simulink library "vmc"  (R2021b)
settings: Solver=VariableStepAuto  StartTime=0.0  StopTime=10.0  RelTol=1e-3
undefined symbols (not defined in the file): AVMC_ACCDeltaTqGradeGn_X_deg, AVMC_ACCDeltaTqIGain4OVRD_X_kph, AVMC_ACCDeltaTqIGain4OVRD_Y_mps2, AVMC_ACCDeltaTqIGain_X_kph, AVMC_ACCDeltaTqIGain_Y_mps2, AVMC_ACCDeltaTqPGain_X_kph, AVMC_ACCDeltaTqPGain_Y_kph, AVMC_ACCGradeofst_X_G, AVMC_ACCGradeofst_Y_pct, AVMC_ACCLoSpdTqLoLim4JP_X_kph, AVMC_ACCLoSpdTqLoLim4JP_Y_deg, AVMC_ACCLoSpdTqLowerLim_X_kph, AVMC_ACCLoSpdTqLowerLim_Y_deg, AVMC_ACCReqAccelGain_X_mps2, AVMC_ACCReqAccelGain_Y_enum, AVMC_ADSPosGFBDeltaTq_X_kph, AVMC_ADSPosGFBDeltaTq_Y_mps2, AVMC_AggressJerkPCT4AT_X_kph, AVMC_AggressJerkPCT_X_kph, AVMC_AggressLimitPCT4AT_X_kph, AVMC_AggressLimitPCT_X_kph, AVMC_DECGradeofst_X_G, AVMC_DECGradeofst_Y_pct, AVMC_DISCDeltaTqIGain_X_kph, AVMC_DISCDeltaTqIGain_Y_mps2, AVMC_DISCDeltaTqPGain_X_kph, AVMC_DISCDeltaTqPGain_Y_kph, AVMC_EPSForceSelect_X_enum, AVMC_EPSForceSelect_Y_enum, AVMC_EPSForceSelectD21_X_enum, AVMC_EPSForceSelectD21_Y_enum, AVMC_ESCRegenOut_X_kph, AVMC_ESCRegenOut_Y_Deg, AVMC_ESCRegenOutEnSpd_X_Deg, AVMC_EstPitchSlopeTs_X_kph, AVMC_GradeCompFlt_X_kph, AVMC_GyroYBandLo_X_Gps, AVMC_HoldResTq_X_kph, AVMC_ISOAccLimit_X_mps, AVMC_ISODecLimit_X_mps, AVMC_ISOJerk_X_mps, AVMC_LatESCRegenOut_X_kph, AVMC_LatESCRegenOut_Y_Deg, AVMC_LongAccDeadZone_X_kph, AVMC_LongAccFiltTsforP2_X_Gps, AVMC_MCPresBaseTq_X_bar, AVMC_MSAPedalOvrd_X_kph, AVMC_MSASpdBand_X_kph, AVMC_MSATqDownEndTq_X_kph, AVMC_MSATqDownTime_X_kph, AVMC_NegZCHoldTq_X_kph, AVMC_OPDDisSlideRate_X_Deg, AVMC_OVRD2ActSR2FCMCMD_X_mps2, AVMC_PedalTqRWhlRatio_X_Nm, AVMC_PedalTqRWhlRatio_Y_gps, AVMC_PedalTqRWhlSlipGain_X_rat, AVMC_PedalTqRWhlSlipGain_Y_kph, AVMC_PedalTqRWhSTRGGain_X_deg, AVMC_PedalTqRWhSTRGGain_Y_kph, AVMC_PosZCHoldTq_X_kph ... (+593)
libraries: hcu_lib x143, simulink x96, tqr x4, $bdroot x1, simulink_extras x1
(part 17 of 17)

== stateflow chart vmc/VMC/VMC/SafetyControl/WheelSpeedRollingAverage/RollingAverage1 ==
  state LatAccelRollingAverage
    (default) -> (junction 2) : {VVMC_RollAveCount_enum = ONE_INT}
    LatAccelRollingAverage -> (junction 2)
    (junction 2) -> (junction 3) : {VVMC_RFWhlSpeedRollAveRaw_kph = ZERO_FLOAT}
    (junction 3) -> (junction 100) [order 1] : [VVMC_RollAveCount_enum < KVMC_WhlSpdRollAveLevel_enum]
    (junction 3) -> (junction 37) [order 2]
    (junction 100) -> (junction 5) : {% Memory
        |  VVMC_Memory_raw32[VVMC_RollAveCount_enum] = VINP_RFRawWhlSpeed_kph;
        |
        |  % Memory Shift Counter
        |  VVMC_ShiftCount_enum = ONE_INT}
    (junction 5) -> (junction 7) [order 2]
    (junction 5) -> (junction 6) [order 1] : [VVMC_ShiftCount_enum <= VVMC_RollAveCount_enum]
    (junction 7) -> (junction 8) : {% Rolling Average
        |  VVMC_RFWhlSpeedRollAveRaw_kph = VVMC_RFWhlSpeedRollAveRaw_kph / VVMC_RollAveCount_enum;
        |
        |  % Rolling Average Counter
        |  VVMC_RollAveCount_enum++}
    (junction 35) -> (junction 5) : {VVMC_ShiftCount_enum++}
    (junction 6) -> (junction 36) : {% Rolling Average Sum
        |  VVMC_RFWhlSpeedRollAveRaw_kph = VVMC_RFWhlSpeedRollAveRaw_kph + VVMC_Memory_raw32[VVMC_ShiftCount_enum];
        |  }
    (junction 36) -> (junction 35)
    (junction 37) -> (junction 76) [order 1] : [VVMC_RollAveCount_enum == KVMC_WhlSpdRollAveLevel_enum]
    (junction 76) -> (junction 47)
    (junction 37) -> (junction 60) [order 2]
    (junction 78) -> (junction 76)
    (junction 47) -> (junction 30) : {% Memory
        |  VVMC_Memory_raw32[VVMC_RollAveCount_enum] = VINP_RFRawWhlSpeed_kph;
        |
        |  % Memory Shift Counter
        |  VVMC_ShiftCount_enum = ONE_INT;
        | }
    (junction 60) -> (junction 62) [order 1] : [VVMC_RollAveCount_enum > KVMC_WhlSpdRollAveLevel_enum]
    (junction 60) -> (junction 39) [order 2]
    (junction 62) -> (junction 66) : {VVMC_MemoryShiftCount_enum = ONE_INT}
    (junction 30) -> (junction 48) [order 2]
    (junction 30) -> (junction 22) [order 1] : [VVMC_ShiftCount_enum <= VVMC_RollAveCount_enum]
    (junction 48) -> (junction 45) : {% Rolling Average
        |  VVMC_RFWhlSpeedRollAveRaw_kph = VVMC_RFWhlSpeedRollAveRaw_kph / VVMC_RollAveCount_enum;
        |
        |  % Memory Shift Counter
        |  VVMC_ShiftCount_enum = ONE_INT}
    (junction 14) -> (junction 30) : {VVMC_ShiftCount_enum++}
    (junction 22) -> (junction 25) : {% Rolling Average Sum
        |  VVMC_RFWhlSpeedRollAveRaw_kph = VVMC_RFWhlSpeedRollAveRaw_kph + VVMC_Memory_raw32[VVMC_ShiftCount_enum]}
    (junction 66) -> (junction 82) [order 2]
    (junction 66) -> (junction 69) [order 1] : [VVMC_MemoryShiftCount_enum < VVMC_RollAveCount_enum]
    (junction 82) -> (junction 80) : {VVMC_RollAveCount_enum = KVMC_WhlSpdRollAveLevel_enum}
    (junction 73) -> (junction 66) : {VVMC_MemoryShiftCount_enum++}
    (junction 69) -> (junction 71) : {VVMC_Memory_raw32[VVMC_MemoryShiftCount_enum] =...
        |  VVMC_Memory_raw32[VVMC_RollAveCount_enum - KVMC_WhlSpdRollAveLevel_enum + VVMC_MemoryShiftCount_enum]}
    (junction 25) -> (junction 14)
    (junction 71) -> (junction 73)
    (junction 80) -> (junction 78)
    (junction 45) -> (junction 39) [order 2]
    (junction 45) -> (junction 15) [order 1] : [VVMC_ShiftCount_enum < VVMC_RollAveCount_enum]
    (junction 41) -> (junction 45) : { VVMC_ShiftCount_enum++}
    (junction 15) -> (junction 38) : {% Gy Memory Shift
        |  VVMC_Memory_raw32[VVMC_ShiftCount_enum] = VVMC_Memory_raw32[VVMC_ShiftCount_enum + ONE_INT]}
    (junction 38) -> (junction 41)
  data: KVMC_WhlSpdRollAveLevel_enum input uint8; VVMC_ShiftCount_enum local uint8; VVMC_RollAveCount_enum local uint8; VVMC_Memory_raw32 local single size=256; ZERO_FLOAT input single; ONE_INT input uint8; VINP_RFRawWhlSpeed_kph input single; VVMC_MemoryShiftCount_enum local uint8; VVMC_RFWhlSpeedRollAveRaw_kph output single

== stateflow chart vmc/VMC/VMC/SafetyControl/WheelSpeedRollingAverage/RollingAverage2 ==
  state LatAccelRollingAverage
    (default) -> (junction 2) : {VVMC_RollAveCount_enum = ONE_INT}
    LatAccelRollingAverage -> (junction 2)
    (junction 2) -> (junction 3) : {VVMC_LRWhlSpeedRollAveRaw_kph = ZERO_FLOAT}
    (junction 3) -> (junction 100) [order 1] : [VVMC_RollAveCount_enum < KVMC_WhlSpdRollAveLevel_enum]
    (junction 3) -> (junction 37) [order 2]
    (junction 100) -> (junction 5) : {% Memory
        |  VVMC_Memory_raw32[VVMC_RollAveCount_enum] = VINP_LRRawWhlSpeed_kph;
        |
        |  % Memory Shift Counter
        |  VVMC_ShiftCount_enum = ONE_INT}
    (junction 5) -> (junction 7) [order 2]
    (junction 5) -> (junction 6) [order 1] : [VVMC_ShiftCount_enum <= VVMC_RollAveCount_enum]
    (junction 7) -> (junction 8) : {% Rolling Average
        |  VVMC_LRWhlSpeedRollAveRaw_kph = VVMC_LRWhlSpeedRollAveRaw_kph / VVMC_RollAveCount_enum;
        |
        |  % Rolling Average Counter
        |  VVMC_RollAveCount_enum++}
    (junction 35) -> (junction 5) : {VVMC_ShiftCount_enum++}
    (junction 6) -> (junction 36) : {% Rolling Average Sum
        |  VVMC_LRWhlSpeedRollAveRaw_kph = VVMC_LRWhlSpeedRollAveRaw_kph + VVMC_Memory_raw32[VVMC_ShiftCount_enum];
        |  }
    (junction 36) -> (junction 35)
    (junction 37) -> (junction 76) [order 1] : [VVMC_RollAveCount_enum == KVMC_WhlSpdRollAveLevel_enum]
    (junction 76) -> (junction 47)
    (junction 37) -> (junction 60) [order 2]
    (junction 78) -> (junction 76)
    (junction 47) -> (junction 30) : {% Memory
        |  VVMC_Memory_raw32[VVMC_RollAveCount_enum] = VINP_LRRawWhlSpeed_kph;
        |
        |  % Memory Shift Counter
        |  VVMC_ShiftCount_enum = ONE_INT;
        | }
    (junction 60) -> (junction 62) [order 1] : [VVMC_RollAveCount_enum > KVMC_WhlSpdRollAveLevel_enum]
    (junction 60) -> (junction 39) [order 2]
    (junction 62) -> (junction 66) : {VVMC_MemoryShiftCount_enum = ONE_INT}
    (junction 30) -> (junction 48) [order 2]
    (junction 30) -> (junction 22) [order 1] : [VVMC_ShiftCount_enum <= VVMC_RollAveCount_enum]
    (junction 48) -> (junction 45) : {% Rolling Average
        |  VVMC_LRWhlSpeedRollAveRaw_kph = VVMC_LRWhlSpeedRollAveRaw_kph / VVMC_RollAveCount_enum;
        |
        |  % Memory Shift Counter
        |  VVMC_ShiftCount_enum = ONE_INT}
    (junction 14) -> (junction 30) : {VVMC_ShiftCount_enum++}
    (junction 22) -> (junction 25) : {% Rolling Average Sum
        |  VVMC_LRWhlSpeedRollAveRaw_kph = VVMC_LRWhlSpeedRollAveRaw_kph + VVMC_Memory_raw32[VVMC_ShiftCount_enum]}
    (junction 66) -> (junction 82) [order 2]
    (junction 66) -> (junction 69) [order 1] : [VVMC_MemoryShiftCount_enum < VVMC_RollAveCount_enum]
    (junction 82) -> (junction 80) : {VVMC_RollAveCount_enum = KVMC_WhlSpdRollAveLevel_enum}
    (junction 73) -> (junction 66) : {VVMC_MemoryShiftCount_enum++}
    (junction 69) -> (junction 71) : {VVMC_Memory_raw32[VVMC_MemoryShiftCount_enum] =...
        |  VVMC_Memory_raw32[VVMC_RollAveCount_enum - KVMC_WhlSpdRollAveLevel_enum + VVMC_MemoryShiftCount_enum]}
    (junction 25) -> (junction 14)
    (junction 71) -> (junction 73)
    (junction 80) -> (junction 78)
    (junction 45) -> (junction 39) [order 2]
    (junction 45) -> (junction 15) [order 1] : [VVMC_ShiftCount_enum < VVMC_RollAveCount_enum]
    (junction 41) -> (junction 45) : { VVMC_ShiftCount_enum++}
    (junction 15) -> (junction 38) : {% Gy Memory Shift
        |  VVMC_Memory_raw32[VVMC_ShiftCount_enum] = VVMC_Memory_raw32[VVMC_ShiftCount_enum + ONE_INT]}
    (junction 38) -> (junction 41)
  data: KVMC_WhlSpdRollAveLevel_enum input uint8; VVMC_ShiftCount_enum local uint8; VVMC_RollAveCount_enum local uint8; VVMC_Memory_raw32 local single size=256; ZERO_FLOAT input single; ONE_INT input uint8; VINP_LRRawWhlSpeed_kph input single; VVMC_MemoryShiftCount_enum local uint8; VVMC_LRWhlSpeedRollAveRaw_kph output single

== stateflow chart vmc/VMC/VMC/SafetyControl/WheelSpeedRollingAverage/RollingAverage3 ==
  state LatAccelRollingAverage
    (default) -> (junction 2) : {VVMC_RollAveCount_enum = ONE_INT}
    LatAccelRollingAverage -> (junction 2)
    (junction 2) -> (junction 3) : {VVMC_RRWhlSpeedRollAveRaw_kph = ZERO_FLOAT}
    (junction 3) -> (junction 100) [order 1] : [VVMC_RollAveCount_enum < KVMC_WhlSpdRollAveLevel_enum]
    (junction 3) -> (junction 37) [order 2]
    (junction 100) -> (junction 5) : {% Memory
        |  VVMC_Memory_raw32[VVMC_RollAveCount_enum] = VINP_RRRawWhlSpeed_kph;
        |
        |  % Memory Shift Counter
        |  VVMC_ShiftCount_enum = ONE_INT}
    (junction 5) -> (junction 7) [order 2]
    (junction 5) -> (junction 6) [order 1] : [VVMC_ShiftCount_enum <= VVMC_RollAveCount_enum]
    (junction 7) -> (junction 8) : {% Rolling Average
        |  VVMC_RRWhlSpeedRollAveRaw_kph = VVMC_RRWhlSpeedRollAveRaw_kph / VVMC_RollAveCount_enum;
        |
        |  % Rolling Average Counter
        |  VVMC_RollAveCount_enum++}
    (junction 35) -> (junction 5) : {VVMC_ShiftCount_enum++}
    (junction 6) -> (junction 36) : {% Rolling Average Sum
        |  VVMC_RRWhlSpeedRollAveRaw_kph = VVMC_RRWhlSpeedRollAveRaw_kph + VVMC_Memory_raw32[VVMC_ShiftCount_enum];
        |  }
    (junction 36) -> (junction 35)
    (junction 37) -> (junction 76) [order 1] : [VVMC_RollAveCount_enum == KVMC_WhlSpdRollAveLevel_enum]
    (junction 76) -> (junction 47)
    (junction 37) -> (junction 60) [order 2]
    (junction 78) -> (junction 76)
    (junction 47) -> (junction 30) : {% Memory
        |  VVMC_Memory_raw32[VVMC_RollAveCount_enum] = VINP_RRRawWhlSpeed_kph;
        |
        |  % Memory Shift Counter
        |  VVMC_ShiftCount_enum = ONE_INT;
        | }
    (junction 60) -> (junction 62) [order 1] : [VVMC_RollAveCount_enum > KVMC_WhlSpdRollAveLevel_enum]
    (junction 60) -> (junction 39) [order 2]
    (junction 62) -> (junction 66) : {VVMC_MemoryShiftCount_enum = ONE_INT}
    (junction 30) -> (junction 48) [order 2]
    (junction 30) -> (junction 22) [order 1] : [VVMC_ShiftCount_enum <= VVMC_RollAveCount_enum]
    (junction 48) -> (junction 45) : {% Rolling Average
        |  VVMC_RRWhlSpeedRollAveRaw_kph = VVMC_RRWhlSpeedRollAveRaw_kph / VVMC_RollAveCount_enum;
        |
        |  % Memory Shift Counter
        |  VVMC_ShiftCount_enum = ONE_INT}
    (junction 14) -> (junction 30) : {VVMC_ShiftCount_enum++}
    (junction 22) -> (junction 25) : {% Rolling Average Sum
        |  VVMC_RRWhlSpeedRollAveRaw_kph = VVMC_RRWhlSpeedRollAveRaw_kph + VVMC_Memory_raw32[VVMC_ShiftCount_enum]}
    (junction 66) -> (junction 82) [order 2]
    (junction 66) -> (junction 69) [order 1] : [VVMC_MemoryShiftCount_enum < VVMC_RollAveCount_enum]
    (junction 82) -> (junction 80) : {VVMC_RollAveCount_enum = KVMC_WhlSpdRollAveLevel_enum}
    (junction 73) -> (junction 66) : {VVMC_MemoryShiftCount_enum++}
    (junction 69) -> (junction 71) : {VVMC_Memory_raw32[VVMC_MemoryShiftCount_enum] =...
        |  VVMC_Memory_raw32[VVMC_RollAveCount_enum - KVMC_WhlSpdRollAveLevel_enum + VVMC_MemoryShiftCount_enum]}
    (junction 25) -> (junction 14)
    (junction 71) -> (junction 73)
    (junction 80) -> (junction 78)
    (junction 45) -> (junction 39) [order 2]
    (junction 45) -> (junction 15) [order 1] : [VVMC_ShiftCount_enum < VVMC_RollAveCount_enum]
    (junction 41) -> (junction 45) : { VVMC_ShiftCount_enum++}
    (junction 15) -> (junction 38) : {% Gy Memory Shift
        |  VVMC_Memory_raw32[VVMC_ShiftCount_enum] = VVMC_Memory_raw32[VVMC_ShiftCount_enum + ONE_INT]}
    (junction 38) -> (junction 41)
  data: KVMC_WhlSpdRollAveLevel_enum input uint8; VVMC_ShiftCount_enum local uint8; VVMC_RollAveCount_enum local uint8; VVMC_Memory_raw32 local single size=256; ZERO_FLOAT input single; ONE_INT input uint8; VINP_RRRawWhlSpeed_kph input single; VVMC_MemoryShiftCount_enum local uint8; VVMC_RRWhlSpeedRollAveRaw_kph output single

== stateflow chart vmc/VMC/VMC/Scheduler ==
  state Scheduler
    (default) -> (junction 3) : {counter = 0;}
    Scheduler -> (junction 3) : {counter++}
    (junction 3) -> (junction 5) [order 1] : [counter%%2 == 0]
    (junction 3) -> (junction 11) [order 2]
    (junction 5) -> (junction 7) : {Trigger_10ms_1;
        |  counter = 0;}
    (junction 7) -> (junction 11)
  data: counter local uint8
  events: Trigger_10ms_1 output FUNCTION_CALL_EVENT

== stateflow chart vmc/VMC/VMC/SpeedArbitration/Feature Arbitration/Feature Arbitration ==
  state FeatureArbitration
    (default) -> (junction 406) : {VVMC_FeatArbitrSta_enum = ENUM_FEATARBITRSTA_INACTIVE;
        |  VVMC_FeatReqSpd_kph = ZERO_FLOAT;}
    FeatureArbitration -> (junction 406)
    (junction 406) -> (junction 409) [order 1] : [VVMC_FeatStaConfirm_enum == ENUM_FEATSTACFM_AEB]
    (junction 406) -> (junction 413) [order 2]
    (junction 409) -> (junction 411) : {VVMC_FeatArbitrSta_enum = ENUM_FEATARBITRSTA_AEB;
        |  VVMC_FeatReqSpd_kph = ZERO_FLOAT}
    (junction 413) -> (junction 415) [order 1] : [VVMC_FeatStaConfirm_enum == ENUM_FEATSTACFM_ACC]
    (junction 413) -> (junction 430) [order 2]
    (junction 415) -> (junction 417) : {VVMC_FeatArbitrSta_enum = ENUM_FEATARBITRSTA_ACC;
        |  VVMC_FeatReqSpd_kph = ZERO_FLOAT}
    (junction 430) -> (junction 431) [order 1] : [VVMC_FeatStaConfirm_enum == ENUM_FEATSTACFM_CC]
    (junction 430) -> (junction 440) [order 2]
    (junction 431) -> (junction 433) : {VVMC_FeatArbitrSta_enum = ENUM_FEATARBITRSTA_CC;
        |  VVMC_FeatReqSpd_kph = VVMC_FeatSetSpdForCalcu_kph}
    (junction 440) -> (junction 441) [order 1] : [VVMC_FeatStaConfirm_enum == ENUM_FEATSTACFM_DISC]
    (junction 440) -> (junction 445) [order 2]
    (junction 441) -> (junction 438) : {VVMC_FeatArbitrSta_enum = ENUM_FEATARBITRSTA_DISC;
        |  VVMC_FeatReqSpd_kph = VDSC_DISCTargetSpd_kph}
    (junction 445) -> (junction 443) [order 1] : [VVMC_FeatStaConfirm_enum == ENUM_FEATSTACFM_MSA]
    (junction 445) -> (junction 449) [order 2]
    (junction 443) -> (junction 444) : {VVMC_FeatArbitrSta_enum = ENUM_FEATARBITRSTA_MSA;
        |  VVMC_FeatReqSpd_kph = VVMC_FeatSetSpdForCalcu_kph}
    (junction 449) -> (junction 450) [order 1] : [VVMC_FeatStaConfirm_enum == ENUM_FEATSTACFM_ACCDISC]
    (junction 450) -> (junction 557) [order 1] : [VVMC_FeatSetSpdForCalcu_kph < VDSC_DISCTargetSpd_kph &&...
        |  !VDSC_PreACC_flg]
    (junction 449) -> (junction 512) [order 2]
    (junction 450) -> (junction 467) [order 2] : {VVMC_FeatArbitrSta_enum = ENUM_FEATARBITRSTA_ACCDISC;
        |  VVMC_FeatReqSpd_kph = VDSC_DISCTargetSpd_kph}
    (junction 557) -> (junction 553) : {VVMC_FeatArbitrSta_enum = ENUM_FEATARBITRSTA_ACC;
        |  VVMC_FeatReqSpd_kph = ZERO_FLOAT}
    (junction 512) -> (junction 514) [order 1] : [VVMC_FeatStaConfirm_enum == ENUM_FEATSTACFM_CCDISC ||...
        |  VVMC_FeatStaConfirm_enum == ENUM_FEATSTACFM_DISCMSA]
    (junction 514) -> (junction 516) [order 1] : [VVMC_FeatSetSpdForCalcu_kph < VDSC_DISCTargetSpd_kph]
    (junction 516) -> (junction 518) [order 1] : [VVMC_FeatStaConfirm_enum == ENUM_FEATSTACFM_CCDISC]
    (junction 512) -> (junction 527) [order 2] : {VVMC_FeatArbitrSta_enum = ENUM_FEATARBITRSTA_INACTIVE;
        |  VVMC_FeatReqSpd_kph = ZERO_FLOAT}
    (junction 514) -> (junction 525) [order 2] : {VVMC_FeatArbitrSta_enum = ENUM_FEATARBITRSTA_DISC;
        |  VVMC_FeatReqSpd_kph = VDSC_DISCTargetSpd_kph}
    (junction 516) -> (junction 522) [order 2] : {VVMC_FeatArbitrSta_enum = ENUM_FEATARBITRSTA_MSA;
        |  VVMC_FeatReqSpd_kph = VVMC_FeatSetSpdForCalcu_kph}
    (junction 518) -> (junction 520) : {VVMC_FeatArbitrSta_enum = ENUM_FEATARBITRSTA_CC;
        |  VVMC_FeatReqSpd_kph = VVMC_FeatSetSpdForCalcu_kph}
  data: VVMC_FeatStaConfirm_enum input uint8; VDSC_DISCTargetSpd_kph input single; VVMC_FeatSetSpdForCalcu_kph input single; VVMC_FeatArbitrSta_enum output uint8; VVMC_FeatReqSpd_kph output single; ENUM_FEATSTACFM_AEB input uint8; ENUM_FEATSTACFM_ACC input uint8; ENUM_FEATSTACFM_CC input uint8; ENUM_FEATSTACFM_DISC input uint8; ENUM_FEATSTACFM_MSA input uint8; ENUM_FEATSTACFM_ACCDISC input uint8; ENUM_FEATSTACFM_CCDISC input uint8; ENUM_FEATSTACFM_DISCMSA input uint8; ENUM_FEATARBITRSTA_INACTIVE input uint8; ENUM_FEATARBITRSTA_AEB input uint8; ENUM_FEATARBITRSTA_ACC input uint8; ENUM_FEATARBITRSTA_CC input uint8; ENUM_FEATARBITRSTA_DISC input uint8; ENUM_FEATARBITRSTA_ACCDISC input uint8; ENUM_FEATARBITRSTA_MSA input uint8; ZERO_FLOAT input single; VDSC_PreACC_flg input

== stateflow chart vmc/VMC/VMC/SpeedArbitration/Feature Status Confirm/Feature Status Confirm ==
  state FeatStaConfrim
    (default) -> (junction 197) : {VVMC_FeatStaConfirm_enum = ENUM_FEATSTACFM_INACTIVE}
    FeatStaConfrim -> (junction 197)
    (junction 197) -> (junction 203) [order 1] : [VVMC_VMCAEBCtrlAvail_flg == ENUM_VMCAEBCTRLAVAIL_AVAILABLE &&...
        | (VINP_ADASAEBSta_enum == ENUM_ADASAEBSTA_ACTIVE ||...
        |  VINP_ADASAEBReq_enum ~= ENUM_ADASAEBREQ_NOREQUEST)]
    (junction 197) -> (junction 200) [order 2]
    (junction 203) -> (junction 202) : {VVMC_FeatStaConfirm_enum = ENUM_FEATSTACFM_AEB}
    (junction 200) -> (junction 208) [order 1] : [VVMC_VMCACCCtrlAvail_flg == ENUM_VMCACCCTRLAVAIL_AVAILABLE &&...
        | (VDSC_DISCSta_enum == ENUM_DISCSTA_ACTIVE || VDSC_PreACC_flg)]
    (junction 208) -> (junction 210) [order 1] : [VINP_ADASACCSta_enum == ENUM_ADASACCSTA_ACTIVE ||...
        |  VINP_ADASACCSta_enum == ENUM_ADASACCSTA_SHUTOFF ||...
        |  VINP_ADASACCSta_enum == ENUM_ADASACCSTA_OVERRIDE]
    (junction 200) -> (junction 232) [order 2]
    (junction 208) -> (junction 214) [order 2]
    (junction 210) -> (junction 212) : {VVMC_FeatStaConfirm_enum = ENUM_FEATSTACFM_ACCDISC}
    (junction 214) -> (junction 216) [order 1] : [(VVMC_CCCtrlSta_enum == ENUM_CCCRLSTA_ACTIVE ||...
        |   VVMC_CCCtrlSta_enum == ENUM_CCCRLSTA_OVERRIDE) &&...
        |  VVMC_VMCCCCtrlAvail_flg == ENUM_VMCCCCTRLAVAIL_AVAILABLE]
    (junction 214) -> (junction 222) [order 2]
    (junction 216) -> (junction 218) : {VVMC_FeatStaConfirm_enum = ENUM_FEATSTACFM_CCDISC}
    (junction 222) -> (junction 224) [order 1] : [(VVMC_MSACtrlSta_enum == ENUM_MSACRLSTA_ACTIVE ||...
        |   VVMC_MSACtrlSta_enum == ENUM_MSACRLSTA_OVERRIDE) &&...
        |  VVMC_VMCMSACtrlAvail_flg == ENUM_VMCMSACTRLAVAIL_AVAILABLE]
    (junction 222) -> (junction 229) [order 2] : {VVMC_FeatStaConfirm_enum = ENUM_FEATSTACFM_DISC}
    (junction 224) -> (junction 221) : {VVMC_FeatStaConfirm_enum = ENUM_FEATSTACFM_DISCMSA}
    (junction 232) -> (junction 234) [order 1] : [VVMC_VMCACCCtrlAvail_flg == ENUM_VMCACCCTRLAVAIL_AVAILABLE &&...
        | (VINP_ADASACCSta_enum == ENUM_ADASACCSTA_ACTIVE ||...
        |  VINP_ADASACCSta_enum == ENUM_ADASACCSTA_OVERRIDE ||...
        |  VINP_ADASACCSta_enum == ENUM_ADASACCSTA_SHUTOFF)]
    (junction 232) -> (junction 238) [order 2]
    (junction 234) -> (junction 236) : {VVMC_FeatStaConfirm_enum = ENUM_FEATSTACFM_ACC}
    (junction 238) -> (junction 240) [order 1] : [(VVMC_CCCtrlSta_enum == ENUM_CCCRLSTA_ACTIVE ||...
        |   VVMC_CCCtrlSta_enum == ENUM_CCCRLSTA_OVERRIDE) &&...
        |  VVMC_VMCCCCtrlAvail_flg == ENUM_VMCCCCTRLAVAIL_AVAILABLE]
    (junction 238) -> (junction 250) [order 2]
    (junction 240) -> (junction 244) : {VVMC_FeatStaConfirm_enum = ENUM_FEATSTACFM_CC}
    (junction 250) -> (junction 249) [order 1] : [(VVMC_MSACtrlSta_enum == ENUM_MSACRLSTA_ACTIVE ||...
        |   VVMC_MSACtrlSta_enum == ENUM_MSACRLSTA_OVERRIDE) &&...
        |  VVMC_VMCMSACtrlAvail_flg == ENUM_VMCMSACTRLAVAIL_AVAILABLE]
    (junction 250) -> (junction 252) [order 2] : {VVMC_FeatStaConfirm_enum = ENUM_FEATSTACFM_INACTIVE}
    (junction 249) -> (junction 248) : {VVMC_FeatStaConfirm_enum = ENUM_FEATSTACFM_MSA}
  data: VVMC_VMCCCCtrlAvail_flg input boolean; ENUM_VMCCCCTRLAVAIL_AVAILABLE input uint8; VVMC_VMCMSACtrlAvail_flg input boolean; ENUM_VMCMSACTRLAVAIL_AVAILABLE input uint8; VVMC_VMCAEBCtrlAvail_flg input boolean; ENUM_VMCAEBCTRLAVAIL_AVAILABLE input uint8; VVMC_VMCACCCtrlAvail_flg input boolean; ENUM_VMCACCCTRLAVAIL_AVAILABLE input uint8; VINP_ADASAEBSta_enum input uint8; VDSC_DISCSta_enum input uint8; VINP_ADASACCSta_enum input uint8; VVMC_CCCtrlSta_enum input uint8; VVMC_FeatStaConfirm_enum output uint8; VVMC_MSACtrlSta_enum input uint8; ENUM_FEATSTACFM_INACTIVE input uint8; ENUM_FEATSTACFM_AEB input uint8; ENUM_FEATSTACFM_ACC input uint8; ENUM_FEATSTACFM_CC input uint8; ENUM_FEATSTACFM_DISC input uint8; ENUM_FEATSTACFM_MSA input uint8; ENUM_FEATSTACFM_ACCDISC input uint8; ENUM_FEATSTACFM_CCDISC input uint8; ENUM_FEATSTACFM_DISCMSA input uint8; ENUM_ADASAEBSTA_ACTIVE input uint8; ENUM_ADASACCSTA_ACTIVE input uint8; ENUM_ADASACCSTA_SHUTOFF input uint8; ENUM_CCCRLSTA_ACTIVE input uint8; ENUM_MSACRLSTA_ACTIVE input uint8; ENUM_DISCSTA_ACTIVE input uint8; ENUM_ADASACCSTA_OVERRIDE input uint8; VINP_ADASAEBReq_enum input uint8; ENUM_ADASAEBREQ_NOREQUEST input uint8; ENUM_CCCRLSTA_OVERRIDE input; ENUM_MSACRLSTA_OVERRIDE input; VDSC_PreACC_flg input

== stateflow chart vmc/VMC/VMC/SpeedArbitration/Response Gain/Response Gain ==
  state ResponseGain
    (default) -> (junction 81) : {VVMC_JerkPCT_pct = ZERO_FLOAT;
        |  VVMC_LimitPCT_pct = ZERO_FLOAT}
    ResponseGain -> (junction 81)
    (junction 81) -> (junction 73) [order 1] : [VVMC_FeatArbitrSta_enum == ENUM_FEATARBITRSTA_DISC ||...
        |  VVMC_FeatArbitrSta_enum == ENUM_FEATARBITRSTA_CC ||...
        |  VVMC_FeatArbitrSta_enum == ENUM_FEATARBITRSTA_MSA ||...
        |  VVMC_FeatArbitrSta_enum == ENUM_FEATARBITRSTA_ACCDISC]
    (junction 73) -> (junction 75) [order 1] : [VDSC_DISCTurn_flg == ENUM_DISCTURN_ACTIVE ||...
        | (VVMC_FeatArbitrSta_enum == ENUM_FEATARBITRSTA_MSA &&...
        |  KVMC_MSAResponseAGSV_flg == TRUE)]
    (junction 81) -> (junction 92) [order 2] : {VVMC_JerkPCT_pct = ZERO_FLOAT;
        |  VVMC_LimitPCT_pct = ZERO_FLOAT}
    (junction 73) -> (junction 77) [order 2] : {VVMC_JerkPCT_pct = VVMC_SoftJerkPCT_pct;
        |  VVMC_LimitPCT_pct = VVMC_SoftLimitPCT_pct}
    (junction 75) -> (junction 78) : {VVMC_JerkPCT_pct = VVMC_AggressJerkPCT_pct;
        |  VVMC_LimitPCT_pct = VVMC_AggressLimitPCT_pct}
  data: VDSC_DISCTurn_flg input uint8; VVMC_FeatArbitrSta_enum input uint8; VVMC_JerkPCT_pct output single; VVMC_LimitPCT_pct output single; VVMC_SoftJerkPCT_pct input single; VVMC_AggressJerkPCT_pct input single; VVMC_SoftLimitPCT_pct input single; VVMC_AggressLimitPCT_pct input single; ENUM_FEATARBITRSTA_DISC input uint8; ENUM_FEATARBITRSTA_CC input; ZERO_FLOAT input single; ENUM_DISCTURN_ACTIVE input uint8; ENUM_FEATARBITRSTA_ACCDISC input uint8; ENUM_FEATARBITRSTA_MSA input; TRUE input; KVMC_MSAResponseAGSV_flg input; ENUM_FEATARBITRSTA_ACC parameter

== stateflow chart vmc/VMC/VMC/SpeedCalculation/RollingAverage ==
  state LatAccelRollingAverage
    (default) -> (junction 2) : {VVMC_RollAveCount_enum = ONE_INT}
    LatAccelRollingAverage -> (junction 2)
    (junction 2) -> (junction 3) : {VVMC_RollAve_kph = ZERO_FLOAT}
    (junction 3) -> (junction 100) [order 1] : [VVMC_RollAveCount_enum < KVMC_RollAveLevel_enum]
    (junction 3) -> (junction 37) [order 2]
    (junction 100) -> (junction 5) : {% Memory
        |  VVMC_Memory_raw32[VVMC_RollAveCount_enum] = VINP_RawData_kph;
        |
        |  % Memory Shift Counter
        |  VVMC_ShiftCount_enum = ONE_INT}
    (junction 5) -> (junction 7) [order 2]
    (junction 5) -> (junction 6) [order 1] : [VVMC_ShiftCount_enum <= VVMC_RollAveCount_enum]
    (junction 7) -> (junction 8) : {% Rolling Average
        |  VVMC_RollAve_kph = VVMC_RollAve_kph / VVMC_RollAveCount_enum;
        |
        |  % Rolling Average Counter
        |  VVMC_RollAveCount_enum++}
    (junction 35) -> (junction 5) : {VVMC_ShiftCount_enum++}
    (junction 6) -> (junction 36) : {% Rolling Average Sum
        |  VVMC_RollAve_kph = VVMC_RollAve_kph + VVMC_Memory_raw32[VVMC_ShiftCount_enum];
        |  }
    (junction 36) -> (junction 35)
    (junction 37) -> (junction 76) [order 1] : [VVMC_RollAveCount_enum == KVMC_RollAveLevel_enum]
    (junction 76) -> (junction 47)
    (junction 37) -> (junction 60) [order 2]
    (junction 78) -> (junction 76)
    (junction 47) -> (junction 30) : {% Memory
        |  VVMC_Memory_raw32[VVMC_RollAveCount_enum] = VINP_RawData_kph;
        |
        |  % Memory Shift Counter
        |  VVMC_ShiftCount_enum = ONE_INT;
        | }
    (junction 60) -> (junction 62) [order 1] : [VVMC_RollAveCount_enum > KVMC_RollAveLevel_enum]
    (junction 60) -> (junction 39) [order 2]
    (junction 62) -> (junction 66) : {VVMC_MemoryShiftCount_enum = ONE_INT}
    (junction 30) -> (junction 48) [order 2]
    (junction 30) -> (junction 22) [order 1] : [VVMC_ShiftCount_enum <= VVMC_RollAveCount_enum]
    (junction 48) -> (junction 45) : {% Rolling Average
        |  VVMC_RollAve_kph = VVMC_RollAve_kph / VVMC_RollAveCount_enum;
        |
        |  % Memory Shift Counter
        |  VVMC_ShiftCount_enum = ONE_INT}
    (junction 14) -> (junction 30) : {VVMC_ShiftCount_enum++}
    (junction 22) -> (junction 25) : {% Rolling Average Sum
        |  VVMC_RollAve_kph = VVMC_RollAve_kph + VVMC_Memory_raw32[VVMC_ShiftCount_enum]}
    (junction 66) -> (junction 82) [order 2]
    (junction 66) -> (junction 69) [order 1] : [VVMC_MemoryShiftCount_enum < VVMC_RollAveCount_enum]
    (junction 82) -> (junction 80) : {VVMC_RollAveCount_enum = KVMC_RollAveLevel_enum}
    (junction 73) -> (junction 66) : {VVMC_MemoryShiftCount_enum++}
    (junction 69) -> (junction 71) : {VVMC_Memory_raw32[VVMC_MemoryShiftCount_enum] =...
        |  VVMC_Memory_raw32[VVMC_RollAveCount_enum - KVMC_RollAveLevel_enum + VVMC_MemoryShiftCount_enum]}
    (junction 25) -> (junction 14)
    (junction 71) -> (junction 73)
    (junction 80) -> (junction 78)
    (junction 45) -> (junction 39) [order 2]
    (junction 45) -> (junction 15) [order 1] : [VVMC_ShiftCount_enum < VVMC_RollAveCount_enum]
    (junction 41) -> (junction 45) : { VVMC_ShiftCount_enum++}
    (junction 15) -> (junction 38) : {% Gy Memory Shift
        |  VVMC_Memory_raw32[VVMC_ShiftCount_enum] = VVMC_Memory_raw32[VVMC_ShiftCount_enum + ONE_INT]}
    (junction 38) -> (junction 41)
  data: KVMC_RollAveLevel_enum input uint8; VVMC_ShiftCount_enum local uint8; VVMC_RollAveCount_enum local uint8; VVMC_Memory_raw32 local single size=256; ZERO_FLOAT input single; ONE_INT input uint8; VVMC_RollAve_kph output single; VINP_RawData_kph input single; VVMC_MemoryShiftCount_enum local uint8

== stateflow chart vmc/VMC/VMC/Scheduler1 ==
  state Scheduler
    (default) -> (junction 3) : {counter = 0;}
    Scheduler -> (junction 3) : {counter++}
    (junction 3) -> (junction 5) [order 1] : [counter%%2 == 0]
    (junction 3) -> (junction 11) [order 2]
    (junction 5) -> (junction 7) : {Trigger_LongAccel;
        |  counter = 0;}
    (junction 7) -> (junction 11)
  data: counter local uint8
  events: Trigger_LongAccel output FUNCTION_CALL_EVENT

== stateflow chart vmc/VMC/VMC/ACC_Function/ACC Torque Source Determination/TimeGapJudgement ==
  state TimeGapJudgement
    (default) -> (junction 11) : {VVMC_TimeGapJudge_flag = FALSE}
    TimeGapJudgement -> (junction 11)
    (junction 11) -> (junction 71) [order 1] : [(VVMC_VehicleSpeed_kph * KPH2MPS) > ZERO_FLOAT]
    (junction 11) -> (junction 33) [order 2] : {VVMC_TimeGapJudge_flag = FALSE;
        |  VVMC_TimeGapCalcu_s = KVMC_TimeGapMax_s}
    (junction 71) -> (junction 24) : {VVMC_TimeGapCalcu_s = VINP_ACCObjDist_m / (VVMC_VehicleSpeed_kph * KPH2MPS)}
    (junction 24) -> (junction 29) [order 1] : [VINP_TimeGapLevel_enum == ENUM_TIMEGAPLEVEL_LEVEL1]
    (junction 29) -> (junction 27) [order 1] : [VVMC_TimeGapCalcu_s <= KVMC_TimeGapBandLv1_s]
    (junction 24) -> (junction 35) [order 2]
    (junction 29) -> (junction 44) [order 2] : {VVMC_TimeGapJudge_flag = FALSE}
    (junction 27) -> (junction 31) : {VVMC_TimeGapJudge_flag = TRUE}
    (junction 35) -> (junction 38) [order 1] : [VINP_TimeGapLevel_enum == ENUM_TIMEGAPLEVEL_LEVEL2]
    (junction 38) -> (junction 42) [order 1] : [VVMC_TimeGapCalcu_s <= KVMC_TimeGapBandLv2_s]
    (junction 35) -> (junction 56) [order 2]
    (junction 38) -> (junction 46) [order 2] : {VVMC_TimeGapJudge_flag = FALSE}
    (junction 42) -> (junction 40) : {VVMC_TimeGapJudge_flag = TRUE}
    (junction 56) -> (junction 49) [order 1] : [VINP_TimeGapLevel_enum == ENUM_TIMEGAPLEVEL_LEVEL3]
    (junction 49) -> (junction 50) [order 1] : [VVMC_TimeGapCalcu_s <= KVMC_TimeGapBandLv3_s]
    (junction 56) -> (junction 59) [order 2]
    (junction 49) -> (junction 48) [order 2] : {VVMC_TimeGapJudge_flag = FALSE}
    (junction 50) -> (junction 53) : {VVMC_TimeGapJudge_flag = TRUE}
    (junction 59) -> (junction 65) [order 1] : [VINP_TimeGapLevel_enum == ENUM_TIMEGAPLEVEL_LEVEL4]
    (junction 65) -> (junction 64) [order 1] : [VVMC_TimeGapCalcu_s <= KVMC_TimeGapBandLv4_s]
    (junction 59) -> (junction 68) [order 2] : {VVMC_TimeGapJudge_flag = FALSE}
    (junction 65) -> (junction 66) [order 2] : {VVMC_TimeGapJudge_flag = FALSE}
    (junction 64) -> (junction 58) : {VVMC_TimeGapJudge_flag = TRUE}
  data: VINP_ACCObjDist_m input single; VVMC_VehicleSpeed_kph input single; KPH2MPS input single; VINP_TimeGapLevel_enum input uint8; VVMC_TimeGapJudge_flag output boolean; ENUM_TIMEGAPLEVEL_LEVEL1 input uint8; KVMC_TimeGapBandLv1_s input single; ENUM_TIMEGAPLEVEL_LEVEL2 input uint8; KVMC_TimeGapBandLv2_s input single; ENUM_TIMEGAPLEVEL_LEVEL3 input uint8; KVMC_TimeGapBandLv3_s input single; ENUM_TIMEGAPLEVEL_LEVEL4 input uint8; KVMC_TimeGapBandLv4_s input single; TRUE input boolean; FALSE input boolean; ZERO_FLOAT input single; KVMC_TimeGapMax_s input single; VVMC_TimeGapCalcu_s output single

== stateflow chart vmc/VMC/VMC/CruiseControlFunction/CCActiveDetermination/Chart ==
  state CCActiveDetermination
    (default) -> (junction 360) : {
        |  VVMC_CCCtrlSta_enum = 0;
        |  VVMC_CCSpdWar_flg = 0;
        |  VVMC_SWCResUpLoop_flg = 0;
        |  VVMC_CruzLoopSpdChk_flg = 0;
        |  VVMC_CheckCmdLoop_flg = 0;
        |  }
    CCActiveDetermination -> (junction 360) [order 4] : {VVMC_SWCResUpLoop_flg = 0;
        |  VVMC_CheckCmdLoop_flg = 0;
        |  VVMC_CruzLoopSpdChk_flg = 0;}
    (junction 360) -> (junction 353) [order 1] : [VTQD_SpdCtrlMode_enum == 2 &&...
        |  VVMC_VMCCCCtrlAvail_flg] %241026
    (junction 353) -> (junction 347) [order 1] : [VTQD_ExternalTqAllow_flg]
    (junction 360) -> (junction 343) [order 2] : {VVMC_CCCtrlSta_enum = 0;}
        | %Phase2 VVMC_CruzActive_flg = 0;}
        | %Back to first loop
        | %add20230706
    (junction 353) -> (junction 367) [order 2] : {VVMC_CCCtrlSta_enum = 5;}
        | %Phase2 VVMC_CruzActive_flg = 0;}
        | %Back to first loop
        | %add20230706
    (junction 347) -> (junction 361) : {VVMC_CCCtrlSta_enum = 1;}
    CCActiveDetermination -> (junction 361) [order 3] : [VVMC_SWCResUpLoop_flg && VTQD_ExternalTqAllow_flg]{VVMC_SWCResUpLoop_flg = 0;} %add20230705 %Phase2 modify
    (junction 361) -> (junction 368) [order 1] : [VVMC_FeatSetSpdFinal_raw32 > ONE_FLOAT &&...
        |  VINP_ADASAEBSta_enum ~= ENUM_ADASAEBSTA_ACTIVE]
    (junction 361) -> (junction 374) [order 2] : %Back to first loop
    (junction 368) -> (junction 344)
    CCActiveDetermination -> (junction 344) [order 1] : [VVMC_CruzLoopSpdChk_flg && VTQD_ExternalTqAllow_flg]{VVMC_CruzLoopSpdChk_flg = 0;} %add20230705
    (junction 344) -> (junction 345) [order 1] : [VVMC_FeatSetSpdFinal_raw32 >= KVMC_CCActiveMetSpdLo_kph &&...
        |  VVMC_FeatSetSpdFinal_raw32 <= KVMC_CCActiveMetSpdHi_kph]
    (junction 344) -> (junction 370) [order 2] : {VVMC_CCSpdWar_flg = 0;}
    (junction 345) -> (junction 375) : %Phase 2 {VVMC_CruzActive_flg = 1;
        | {VVMC_CCCtrlSta_enum = 2;}
    (junction 370) -> (junction 371) [order 1] : [VVMC_FeatSetSpdFinal_raw32 < KVMC_CCActiveMetSpdLo_kph]
    (junction 370) -> (junction 348) [order 2] : {VVMC_CCCtrlSta_enum = 4;}
        | %TBD
    (junction 371) -> (junction 346) : {VVMC_CCCtrlSta_enum = 3;}
        | %TBD
    (junction 346) -> (junction 348)
    (junction 348) -> (junction 355) : {VVMC_SWCResUpLoop_flg = 1;}
    (junction 375) -> (junction 349) [order 1] : [(VVMC_MeterIndSpeed_raw32 - VVMC_FeatSetSpdFinal_raw32) >=...
        |  KVMC_CCMSASpdWar_raw32]
    (junction 375) -> (junction 356) [order 2] : {VVMC_CCSpdWar_flg = 0;}
    (junction 349) -> (junction 363) : {VVMC_CCSpdWar_flg = 1;}
    (junction 363) -> (junction 356)
    (junction 356) -> (junction 376)
    (junction 376) -> (junction 350) [order 1] : [VVMC_CCPedalOvrd_flg]
    (junction 376) -> (junction 351) [order 2] : {VVMC_CCCtrlSta_enum = 2}
    (junction 350) -> (junction 358) : {VVMC_CCCtrlSta_enum = 7}
    (junction 358) -> (junction 351)
    (junction 351) -> (junction 352)
    (junction 352) -> (junction 354) [order 1] : [ VTQD_SpdCtrlMode_enum != 2 ||...
        |   VVMC_DetectSWCCANCEL_flg ||...
        |   VINP_BrkSwSta_flg ||...
        |   VINP_BrakeSWGPIO_flg  ||...
        |   VINP_ADASAEBSta_enum == ENUM_ADASAEBSTA_ACTIVE] %Phase2 add
    (junction 352) -> (junction 357) [order 2] : {VVMC_CruzLoopSpdChk_flg = 1;}
        | %Phase2 modify
    (junction 354) -> (junction 359) : {VVMC_CCSpdWar_flg = 0;}
    CCActiveDetermination -> (junction 359) [order 2] : [VVMC_CheckCmdLoop_flg && VTQD_ExternalTqAllow_flg]{VVMC_CheckCmdLoop_flg = 0;}
    (junction 359) -> (junction 362) [order 1] : [VTQD_SpdCtrlMode_enum == 2 &&...
        |  !VVMC_DetectSWCCANCEL_flg]
    (junction 359) -> (junction 364) [order 2] : %Phase2 {VVMC_CruzActive_flg = 0;
        | {VVMC_CCCtrlSta_enum = 0;}
        | %Back to first loop
    (junction 362) -> (junction 365) : %Phase 2 {VVMC_CruzActive_flg = 0;
        | {VVMC_CCCtrlSta_enum = 1;
        |  VVMC_SWCSetDownLoop_flg = 1;} %Phase2 add
    (junction 365) -> (junction 432) [order 1] : [VVMC_DetectSWCResUp_flg == 1 ||...
        |  VVMC_DetectSWCSetDown_flg == 1]
        | %Phase2 add
    (junction 365) -> (junction 431) [order 2] : {VVMC_CheckCmdLoop_flg = 1}
    (junction 432) -> (junction 433) : {VVMC_SWCResUpLoop_flg = 1}
        | %Phase2 add
  CCActiveDetermination -> CCActiveDetermination [order 1] : [!VTQD_ExternalTqAllow_flg || VTQD_GearActualPosn_enum ~= ENUM_GEARACTUALPOSN_D || !VTQD_ExtDoorAllow_flg || !VVMC_VMCCCCtrlAvail_flg]
      | %add20240918
  data: VVMC_CCCtrlSta_enum output uint8; VTQD_SpdCtrlMode_enum input uint8; VVMC_CCSpdWar_flg output boolean; VTQD_ExternalTqAllow_flg input boolean; VVMC_DetectSWCSetDown_flg input boolean; KVMC_CCActiveMetSpdHi_kph input single; KVMC_CCActiveMetSpdLo_kph input single; VVMC_FeatSetSpdFinal_raw32 input single; KVMC_CCMSASpdWar_raw32 input single; VINP_BrakeSWGPIO_flg input boolean; VVMC_DetectSWCCANCEL_flg input boolean; VINP_BrkSwSta_flg input boolean; VVMC_DetectSWCResUp_flg input boolean; VVMC_CruzLoopSpdChk_flg local boolean; VVMC_SWCSetDownLoop_flg local boolean; VINP_ADASAEBSta_enum input uint8; ENUM_ADASAEBSTA_ACTIVE input uint8; VVMC_CCPedalOvrd_flg input boolean; VTQD_GearActualPosn_enum input uint8; ENUM_GEARACTUALPOSN_D input uint8; VVMC_CheckCmdLoop_flg local boolean; VVMC_SWCResUpLoop_flg local boolean; ONE_FLOAT parameter; VTQD_ExtDoorAllow_flg input; VVMC_VMCCCCtrlAvail_flg input; VVMC_MeterIndSpeed_raw32 input

== stateflow chart vmc/VMC/VMC/FeatureSetSpeed/SpeedDetermination ==
  state SpeedDetermination
    (default) -> (junction 9) : {VVMC_FeatSetSpdFinal_raw32 = ZERO_FLOAT}
    SpeedDetermination -> (junction 9)
    (junction 9) -> (junction 14) [order 1] : [VVMC_APPSpdLimit_flg == ENUM_APPSPDLIMIT_ON]
    (junction 14) -> (junction 16) [order 1] : [VTQD_SpdCtrlSta_flg == ENUM_SCPCRLSTA_ON]
    (junction 9) -> (junction 22) [order 2]
    (junction 14) -> (junction 20) [order 2] : {VVMC_FeatSetSpdFinal_raw32 = VVMC_APPSpdLimit_kph}
    (junction 16) -> (junction 18) : {VVMC_FeatSetSpdFinal_raw32 =...
        |  min(VVMC_APPSpdLimit_kph, VTQD_SetSpd_kph)}
    (junction 22) -> (junction 24) [order 1] : [VTQD_SpdCtrlSta_flg == ENUM_SCPCRLSTA_ON]
    (junction 22) -> (junction 28) [order 2] : {VVMC_FeatSetSpdFinal_raw32 = ZERO_FLOAT}
    (junction 24) -> (junction 26) : {VVMC_FeatSetSpdFinal_raw32 = VTQD_SetSpd_kph}
  data: VVMC_APPSpdLimit_flg input boolean; VTQD_SpdCtrlSta_flg input boolean; VVMC_APPSpdLimit_kph input single; VTQD_SetSpd_kph input single; ENUM_SCPCRLSTA_ON input uint8; ENUM_APPSPDLIMIT_ON input uint8; VVMC_FeatSetSpdFinal_raw32 output single; ZERO_FLOAT input single

== stateflow chart vmc/VMC/VMC/IMU/IMU sensing result /RollingAverage ==
  state RollingAverage
    (default) -> (junction 2) : {VVMC_RollAveCount_enum = ONE_INT}
    RollingAverage -> (junction 2)
    (junction 2) -> (junction 3) : {VVMC_RollAve_raw32 = ZERO_FLOAT}
    (junction 3) -> (junction 100) [order 1] : [VVMC_RollAveCount_enum < KVMC_RollAveLevel_enum]
    (junction 3) -> (junction 37) [order 2]
    (junction 100) -> (junction 5) : {% Memory
        |  VVMC_Memory_raw32[VVMC_RollAveCount_enum] = VINP_INPData_raw32;
        |
        |  % Memory Shift Counter
        |  VVMC_ShiftCount_enum = ONE_INT}
    (junction 5) -> (junction 7) [order 2]
    (junction 5) -> (junction 6) [order 1] : [VVMC_ShiftCount_enum <= VVMC_RollAveCount_enum]
    (junction 7) -> (junction 8) : {% Rolling Average
        |  VVMC_RollAve_raw32 = VVMC_RollAve_raw32 / VVMC_RollAveCount_enum;
        |
        |  % Rolling Average Counter
        |  VVMC_RollAveCount_enum++}
    (junction 35) -> (junction 5) : {VVMC_ShiftCount_enum++}
    (junction 6) -> (junction 36) : {% Rolling Average Sum
        |  VVMC_RollAve_raw32 = VVMC_RollAve_raw32 + VVMC_Memory_raw32[VVMC_ShiftCount_enum];
        |  }
    (junction 36) -> (junction 35)
    (junction 37) -> (junction 76) [order 1] : [VVMC_RollAveCount_enum == KVMC_RollAveLevel_enum]
    (junction 76) -> (junction 47)
    (junction 37) -> (junction 60) [order 2]
    (junction 78) -> (junction 76)
    (junction 47) -> (junction 30) : {% Memory
        |  VVMC_Memory_raw32[VVMC_RollAveCount_enum] = VINP_INPData_raw32;
        |
        |  % Memory Shift Counter
        |  VVMC_ShiftCount_enum = ONE_INT;
        | }
    (junction 60) -> (junction 62) [order 1] : [VVMC_RollAveCount_enum > KVMC_RollAveLevel_enum]
    (junction 60) -> (junction 39) [order 2]
    (junction 62) -> (junction 66) : {VVMC_MemoryShiftCount_enum = ONE_INT}
    (junction 30) -> (junction 48) [order 2]
    (junction 30) -> (junction 22) [order 1] : [VVMC_ShiftCount_enum <= VVMC_RollAveCount_enum]
    (junction 48) -> (junction 45) : {% Rolling Average
        |  VVMC_RollAve_raw32 = VVMC_RollAve_raw32 / VVMC_RollAveCount_enum;
        |
        |  % Memory Shift Counter
        |  VVMC_ShiftCount_enum = ONE_INT}
    (junction 14) -> (junction 30) : {VVMC_ShiftCount_enum++}
    (junction 22) -> (junction 25) : {% Rolling Average Sum
        |  VVMC_RollAve_raw32 = VVMC_RollAve_raw32 + VVMC_Memory_raw32[VVMC_ShiftCount_enum]}
    (junction 66) -> (junction 82) [order 2]
    (junction 66) -> (junction 69) [order 1] : [VVMC_MemoryShiftCount_enum < VVMC_RollAveCount_enum]
    (junction 82) -> (junction 80) : {VVMC_RollAveCount_enum = KVMC_RollAveLevel_enum}
    (junction 73) -> (junction 66) : {VVMC_MemoryShiftCount_enum++}
    (junction 69) -> (junction 71) : {VVMC_Memory_raw32[VVMC_MemoryShiftCount_enum] =...
        |  VVMC_Memory_raw32[VVMC_RollAveCount_enum - KVMC_RollAveLevel_enum + VVMC_MemoryShiftCount_enum]}
    (junction 25) -> (junction 14)
    (junction 71) -> (junction 73)
    (junction 80) -> (junction 78)
    (junction 45) -> (junction 39) [order 2]
    (junction 45) -> (junction 15) [order 1] : [VVMC_ShiftCount_enum < VVMC_RollAveCount_enum]
    (junction 41) -> (junction 45) : { VVMC_ShiftCount_enum++}
    (junction 15) -> (junction 38) : {% Gy Memory Shift
        |  VVMC_Memory_raw32[VVMC_ShiftCount_enum] = VVMC_Memory_raw32[VVMC_ShiftCount_enum + ONE_INT]}
    (junction 38) -> (junction 41)
  data: KVMC_RollAveLevel_enum input uint8; VVMC_ShiftCount_enum local uint8; VVMC_RollAveCount_enum local uint8; VVMC_Memory_raw32 local single size=256; ZERO_FLOAT input single; ONE_INT input uint8; VVMC_RollAve_raw32 output single; VINP_INPData_raw32 input single; VVMC_MemoryShiftCount_enum local uint8

== stateflow chart vmc/VMC/VMC/IMU/IMU sensing result /RollingAverage1 ==
  state RollingAverage
    (default) -> (junction 2) : {VVMC_RollAveCount_enum = ONE_INT}
    RollingAverage -> (junction 2)
    (junction 2) -> (junction 3) : {VVMC_RollAve_raw32 = ZERO_FLOAT}
    (junction 3) -> (junction 100) [order 1] : [VVMC_RollAveCount_enum < KVMC_RollAveLevel_enum]
    (junction 3) -> (junction 37) [order 2]
    (junction 100) -> (junction 5) : {% Memory
        |  VVMC_Memory_raw32[VVMC_RollAveCount_enum] = VINP_INPData_raw32;
        |
        |  % Memory Shift Counter
        |  VVMC_ShiftCount_enum = ONE_INT}
    (junction 5) -> (junction 7) [order 2]
    (junction 5) -> (junction 6) [order 1] : [VVMC_ShiftCount_enum <= VVMC_RollAveCount_enum]
    (junction 7) -> (junction 8) : {% Rolling Average
        |  VVMC_RollAve_raw32 = VVMC_RollAve_raw32 / VVMC_RollAveCount_enum;
        |
        |  % Rolling Average Counter
        |  VVMC_RollAveCount_enum++}
    (junction 35) -> (junction 5) : {VVMC_ShiftCount_enum++}
    (junction 6) -> (junction 36) : {% Rolling Average Sum
        |  VVMC_RollAve_raw32 = VVMC_RollAve_raw32 + VVMC_Memory_raw32[VVMC_ShiftCount_enum];
        |  }
    (junction 36) -> (junction 35)
    (junction 37) -> (junction 76) [order 1] : [VVMC_RollAveCount_enum == KVMC_RollAveLevel_enum]
    (junction 76) -> (junction 47)
    (junction 37) -> (junction 60) [order 2]
    (junction 78) -> (junction 76)
    (junction 47) -> (junction 30) : {% Memory
        |  VVMC_Memory_raw32[VVMC_RollAveCount_enum] = VINP_INPData_raw32;
        |
        |  % Memory Shift Counter
        |  VVMC_ShiftCount_enum = ONE_INT;
        | }
    (junction 60) -> (junction 62) [order 1] : [VVMC_RollAveCount_enum > KVMC_RollAveLevel_enum]
    (junction 60) -> (junction 39) [order 2]
    (junction 62) -> (junction 66) : {VVMC_MemoryShiftCount_enum = ONE_INT}
    (junction 30) -> (junction 48) [order 2]
    (junction 30) -> (junction 22) [order 1] : [VVMC_ShiftCount_enum <= VVMC_RollAveCount_enum]
    (junction 48) -> (junction 45) : {% Rolling Average
        |  VVMC_RollAve_raw32 = VVMC_RollAve_raw32 / VVMC_RollAveCount_enum;
        |
        |  % Memory Shift Counter
        |  VVMC_ShiftCount_enum = ONE_INT}
    (junction 14) -> (junction 30) : {VVMC_ShiftCount_enum++}
    (junction 22) -> (junction 25) : {% Rolling Average Sum
        |  VVMC_RollAve_raw32 = VVMC_RollAve_raw32 + VVMC_Memory_raw32[VVMC_ShiftCount_enum]}
    (junction 66) -> (junction 82) [order 2]
    (junction 66) -> (junction 69) [order 1] : [VVMC_MemoryShiftCount_enum < VVMC_RollAveCount_enum]
    (junction 82) -> (junction 80) : {VVMC_RollAveCount_enum = KVMC_RollAveLevel_enum}
    (junction 73) -> (junction 66) : {VVMC_MemoryShiftCount_enum++}
    (junction 69) -> (junction 71) : {VVMC_Memory_raw32[VVMC_MemoryShiftCount_enum] =...
        |  VVMC_Memory_raw32[VVMC_RollAveCount_enum - KVMC_RollAveLevel_enum + VVMC_MemoryShiftCount_enum]}
    (junction 25) -> (junction 14)
    (junction 71) -> (junction 73)
    (junction 80) -> (junction 78)
    (junction 45) -> (junction 39) [order 2]
    (junction 45) -> (junction 15) [order 1] : [VVMC_ShiftCount_enum < VVMC_RollAveCount_enum]
    (junction 41) -> (junction 45) : { VVMC_ShiftCount_enum++}
    (junction 15) -> (junction 38) : {% Gy Memory Shift
        |  VVMC_Memory_raw32[VVMC_ShiftCount_enum] = VVMC_Memory_raw32[VVMC_ShiftCount_enum + ONE_INT]}
    (junction 38) -> (junction 41)
  data: KVMC_RollAveLevel_enum input uint8; VVMC_ShiftCount_enum local uint8; VVMC_RollAveCount_enum local uint8; VVMC_Memory_raw32 local single size=256; ZERO_FLOAT input single; ONE_INT input uint8; VVMC_RollAve_raw32 output single; VINP_INPData_raw32 input single; VVMC_MemoryShiftCount_enum local uint8

== stateflow chart vmc/VMC/VMC/IMU/IMU sensing result /RollingAverage2 ==
  state RollingAverage
    (default) -> (junction 2) : {VVMC_RollAveCount_enum = ONE_INT}
    RollingAverage -> (junction 2)
    (junction 2) -> (junction 3) : {VVMC_RollAve_raw32 = ZERO_FLOAT}
    (junction 3) -> (junction 100) [order 1] : [VVMC_RollAveCount_enum < KVMC_RollAveLevel_enum]
    (junction 3) -> (junction 37) [order 2]
    (junction 100) -> (junction 5) : {% Memory
        |  VVMC_Memory_raw32[VVMC_RollAveCount_enum] = VINP_INPData_raw32;
        |
        |  % Memory Shift Counter
        |  VVMC_ShiftCount_enum = ONE_INT}
    (junction 5) -> (junction 7) [order 2]
    (junction 5) -> (junction 6) [order 1] : [VVMC_ShiftCount_enum <= VVMC_RollAveCount_enum]
    (junction 7) -> (junction 8) : {% Rolling Average
        |  VVMC_RollAve_raw32 = VVMC_RollAve_raw32 / VVMC_RollAveCount_enum;
        |
        |  % Rolling Average Counter
        |  VVMC_RollAveCount_enum++}
    (junction 35) -> (junction 5) : {VVMC_ShiftCount_enum++}
    (junction 6) -> (junction 36) : {% Rolling Average Sum
        |  VVMC_RollAve_raw32 = VVMC_RollAve_raw32 + VVMC_Memory_raw32[VVMC_ShiftCount_enum];
        |  }
    (junction 36) -> (junction 35)
    (junction 37) -> (junction 76) [order 1] : [VVMC_RollAveCount_enum == KVMC_RollAveLevel_enum]
    (junction 76) -> (junction 47)
    (junction 37) -> (junction 60) [order 2]
    (junction 78) -> (junction 76)
    (junction 47) -> (junction 30) : {% Memory
        |  VVMC_Memory_raw32[VVMC_RollAveCount_enum] = VINP_INPData_raw32;
        |
        |  % Memory Shift Counter
        |  VVMC_ShiftCount_enum = ONE_INT;
        | }
    (junction 60) -> (junction 62) [order 1] : [VVMC_RollAveCount_enum > KVMC_RollAveLevel_enum]
    (junction 60) -> (junction 39) [order 2]
    (junction 62) -> (junction 66) : {VVMC_MemoryShiftCount_enum = ONE_INT}
    (junction 30) -> (junction 48) [order 2]
    (junction 30) -> (junction 22) [order 1] : [VVMC_ShiftCount_enum <= VVMC_RollAveCount_enum]
    (junction 48) -> (junction 45) : {% Rolling Average
        |  VVMC_RollAve_raw32 = VVMC_RollAve_raw32 / VVMC_RollAveCount_enum;
        |
        |  % Memory Shift Counter
        |  VVMC_ShiftCount_enum = ONE_INT}
    (junction 14) -> (junction 30) : {VVMC_ShiftCount_enum++}
    (junction 22) -> (junction 25) : {% Rolling Average Sum
        |  VVMC_RollAve_raw32 = VVMC_RollAve_raw32 + VVMC_Memory_raw32[VVMC_ShiftCount_enum]}
    (junction 66) -> (junction 82) [order 2]
    (junction 66) -> (junction 69) [order 1] : [VVMC_MemoryShiftCount_enum < VVMC_RollAveCount_enum]
    (junction 82) -> (junction 80) : {VVMC_RollAveCount_enum = KVMC_RollAveLevel_enum}
    (junction 73) -> (junction 66) : {VVMC_MemoryShiftCount_enum++}
    (junction 69) -> (junction 71) : {VVMC_Memory_raw32[VVMC_MemoryShiftCount_enum] =...
        |  VVMC_Memory_raw32[VVMC_RollAveCount_enum - KVMC_RollAveLevel_enum + VVMC_MemoryShiftCount_enum]}
    (junction 25) -> (junction 14)
    (junction 71) -> (junction 73)
    (junction 80) -> (junction 78)
    (junction 45) -> (junction 39) [order 2]
    (junction 45) -> (junction 15) [order 1] : [VVMC_ShiftCount_enum < VVMC_RollAveCount_enum]
    (junction 41) -> (junction 45) : { VVMC_ShiftCount_enum++}
    (junction 15) -> (junction 38) : {% Gy Memory Shift
        |  VVMC_Memory_raw32[VVMC_ShiftCount_enum] = VVMC_Memory_raw32[VVMC_ShiftCount_enum + ONE_INT]}
    (junction 38) -> (junction 41)
  data: KVMC_RollAveLevel_enum input uint8; VVMC_ShiftCount_enum local uint8; VVMC_RollAveCount_enum local uint8; VVMC_Memory_raw32 local single size=256; ZERO_FLOAT input single; ONE_INT input uint8; VVMC_RollAve_raw32 output single; VINP_INPData_raw32 input single; VVMC_MemoryShiftCount_enum local uint8
